simulink model "nucleo_g431re_ihm07m1"  (R2024a)
settings: Solver=FixedStepDiscrete  StartTime=0.0  StopTime=10  FixedStep=Ts  RelTol=1e-3  EnableMultiTasking=on
model workspace (MAT data in the model file):
  encoderResolution = 2000
  hallOffset = '0.5'
  indexOffset = 850
  polePairs = '4'
values from neighbouring files (symbols this model uses):
  motorParam =     [matlab.mat]
  PWM_Counter_Period = round(CPU_frequency/PWM_frequency/2)    [mcb_stm32_param_est_InitFunc.m]
  Ts = 1/PWM_frequency    (= 5e-05)    [mcb_stm32_param_est_InitFunc.m]    (also in stm32_pmsm_foc_data.m)
undefined symbols (not defined in the file or in its folder): DiscIntNeverNeededParam, inverter, NumBits1, NumBits2, Slope1, Slope2
libraries: mcbcontrolslib x24, simulink x15, stm32f4xxblockslib x4, stm32g4xxblockslib x3, slpidlib x2, stm32blockslib x2, svdutilitieslib x1
(part 1 of 3)
settings Model: Creator=The MathWorks, Inc.  LastModifiedBy=wsl
settings SolverCC: AlgebraicLoopSolver=TrustRegion  AutoInsertRateTranBlk=on  MaxZcPerStep=1
settings DataIOCC: LimitDataPoints=on  SaveFormat=Array  SaveOutput=off  SaveTime=off  ReturnWorkspaceOutputs=off
settings OptimizationCC: DefaultParameterBehavior=Inlined  DefaultUnderspecifiedDataType=single  InlineInvariantSignals=on  OptimizeBlockIOStorage=off  BufferReuse=off  ReuseModelBlockBuffer=off  GlobalBufferReuse=off  ExpressionFolding=off  ExpressionDepthLimit=2147483647  LocalBlockOutputs=off  ZeroExternalMemoryAtStartup=off  InitFltsAndDblsToZero=on  NoFixptDivByZeroProtection=on  EfficientFloat2IntCast=on  EfficientMapNaN2IntZero=off  LifeSpan=Inf  MaxStackSize=1024  OptimizeDataStoreBuffers=off  BusAssignmentInplaceUpdate=off  EfficientTunableParamExpr=on
settings DebuggingCC: ReadBeforeWriteMsg=DisableAll  WriteAfterWriteMsg=DisableAll  WriteAfterReadMsg=DisableAll  CheckSSInitialOutputMsg=off  SignalResolutionControl=TryResolveAllWithWarning  SolverPrmCheckMsg=warning  InheritedTsInSrcMsg=none  MultiTaskDSMMsg=none  MultiTaskCondExecSysMsg=none  TasksWithSamePriorityMsg=none  SigSpecEnsureSampleTimeMsg=none  IntegerOverflowMsg=none  ParameterPrecisionLossMsg=none  FcnCallInpInsideContextMsg=warning  UnconnectedInputMsg=warning  UnconnectedOutputMsg=warning  UnconnectedLineMsg=warning  AllowSymbolicDim=off  StateNameClashWarn=warning  SubsystemReferenceDiagnosticForUnitTest=warning  SFUnexpectedBacktrackingDiag=warning  SFNoUnconditionalDefaultTransitionDiag=warning  SFExecutionAtInitializationDiag=none  IntegerSaturationMsg=none  ArithmeticOperatorsInVariantConditions=warning
settings HardwareCC: ProdBitPerPointer=32  ProdBitPerSizeT=32  ProdBitPerPtrDiffT=32  ProdLargestAtomicInteger=Long  ProdLargestAtomicFloat=Double  ProdWordSize=32  ProdLongLongMode=on  ProdHWDeviceType=ARM Compatible->ARM Cortex  TargetBitPerChar=16  TargetBitPerInt=16  TargetBitPerPointer=16  TargetLargestAtomicInteger=Integer  TargetIntDivRoundTo=Zero  TargetEndianess=LittleEndian  TargetWordSize=16  TargetHWDeviceType=TI C2000
settings ModelReferenceCC: EnableRefExpFcnMdlSchedulingChecks=on  PropagateSignalLabelsOutOfModel=off
settings SFSimCC: SimUseLocalCustomCode=off  MATLABDynamicMemAlloc=off  CustomCodeUndefinedFunction=UseInterfaceOnly
settings RTWCC: Description=Embedded Coder  SystemTargetFile=ert.tlc  HardwareBoard=STM32G4xx Based  TemplateMakefile=ert_default_tmf  GenerateReport=on  RTWUseLocalCustomCode=off  Toolchain=GNU Tools for ARM Embedded Processors  BuildConfiguration=Faster Runs  IncludeHyperlinkInReport=on  LaunchReport=on  GenerateTraceInfo=on  GenerateTraceReport=on  GenerateTraceReportSl=on  GenerateTraceReportSf=on  GPUComputeCapability=3.5  DLArmComputeVersion=19.05
settings CodeAppCC: IgnoreCustomStorageClasses=off  CustomSymbolStrType=$N$R$M  StateflowObjectComments=on  InternalIdentifier=Classic
settings ERTTargetCC: TargetLangStandard=C99 (ISO)  CodeReplacementLibrary=ARM Cortex-M  MultiwordLength=2048  ExtModeTransport=3  ExtModeStaticAlloc=on  ExtModeStaticAllocSize=2048  ExtModeMexFile=ext_xcp  ExtModeIntrfLevel=Level2 - Open  ConvertIfToSwitch=off  SuppressUnreachableDefaultCases=off  MemSecPackage=tic2000demospkg
settings ConfigComp: CovMetricSettings=dw  CovSaveCumulativeToWorkspaceVar=on  CovSaveSingleToWorkspaceVar=on  CovExternalEMLEnable=off  CovSFcnEnable=off

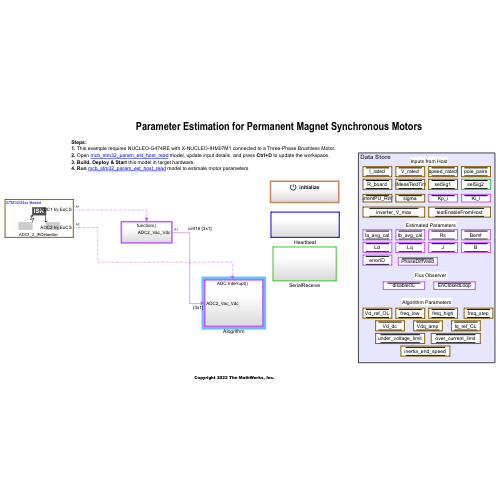
[thumbnail: Simulink's stored preview of the top-level diagram]
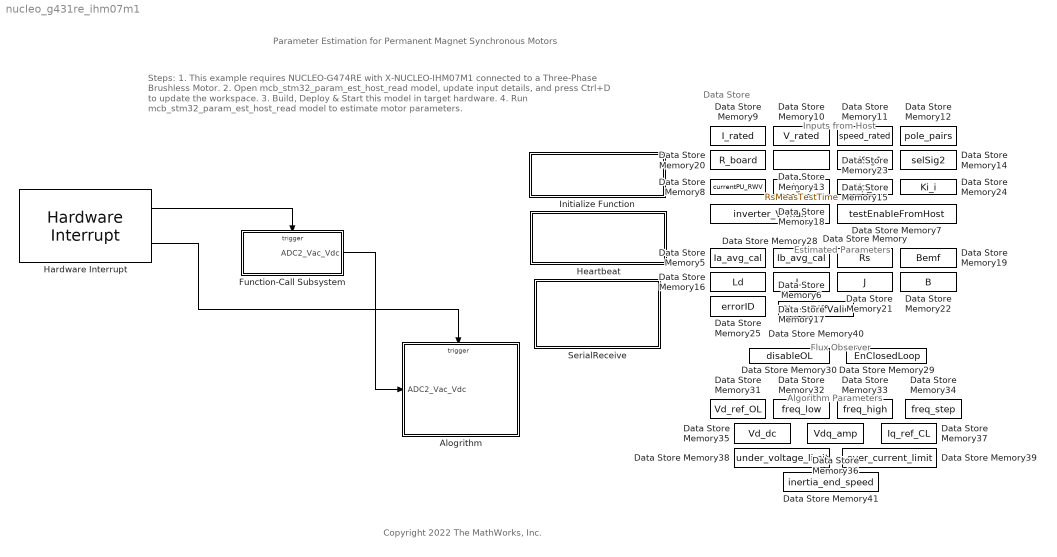
== system nucleo_g431re_ihm07m1 ==
  note: Flux Observer
  note: Estimated Parameters
  note: Data Store
  note: Inputs from Host
  note: Parameter Estimation for Permanent Magnet Synchronous Motors
  note: Steps:
      | 1. This example requires NUCLEO-G474RE with X-NUCLEO-IHM07M1 connected to a Three-Phase Brushless Motor.
      | 2. Open mcb_stm32_param_est_host_read model, update input details, and press Ctrl+D to update the workspace.
      | 3. Build, Deploy & Start this model in target hardware.
      | 4. Run mcb_stm32_param_est_host_read model to estimate motor parameters.
  note: Algorithm Parameters
  note: Copyright 2022 The MathWorks, Inc.
  Alogrithm : Subsystem
  Data Store Memory : DataStoreMemory  DataStoreName=Rs  ReadBeforeWriteMsg=warning  WriteAfterWriteMsg=warning  WriteAfterReadMsg=warning  InitialValue=1  ShowAdditionalParam=off  OutDataTypeStr=single
  Data Store Memory10 : DataStoreMemory  DataStoreName=V_rated  ReadBeforeWriteMsg=warning  WriteAfterWriteMsg=warning  WriteAfterReadMsg=warning  InitialValue=1  ShowAdditionalParam=off  OutDataTypeStr=single
  Data Store Memory11 : DataStoreMemory  DataStoreName=speed_rated  ReadBeforeWriteMsg=warning  WriteAfterWriteMsg=warning  WriteAfterReadMsg=warning  InitialValue=1  ShowAdditionalParam=off  OutDataTypeStr=single
  Data Store Memory12 : DataStoreMemory  DataStoreName=pole_pairs  ReadBeforeWriteMsg=warning  WriteAfterWriteMsg=warning  WriteAfterReadMsg=warning  InitialValue=1  ShowAdditionalParam=off  OutDataTypeStr=single
  Data Store Memory13 : DataStoreMemory  DataStoreName=RsMeasTestTime  ReadBeforeWriteMsg=warning  WriteAfterWriteMsg=warning  WriteAfterReadMsg=warning  InitialValue=1  ShowAdditionalParam=off  OutDataTypeStr=single
  Data Store Memory14 : DataStoreMemory  DataStoreName=selSig2  ReadBeforeWriteMsg=warning  WriteAfterWriteMsg=warning  WriteAfterReadMsg=warning  InitialValue=1  ShowAdditionalParam=off  OutDataTypeStr=single
  Data Store Memory15 : DataStoreMemory  DataStoreName=selSig1  ReadBeforeWriteMsg=warning  WriteAfterWriteMsg=warning  WriteAfterReadMsg=warning  InitialValue=1  ShowAdditionalParam=off  OutDataTypeStr=single
  Data Store Memory16 : DataStoreMemory  DataStoreName=Ld  ReadBeforeWriteMsg=warning  WriteAfterWriteMsg=warning  WriteAfterReadMsg=warning  InitialValue=1  ShowAdditionalParam=off
  Data Store Memory17 : DataStoreMemory  DataStoreName=Lq  ReadBeforeWriteMsg=warning  WriteAfterWriteMsg=warning  WriteAfterReadMsg=warning  InitialValue=1  ShowAdditionalParam=off
  Data Store Memory18 : DataStoreMemory  DataStoreName=sigma  ReadBeforeWriteMsg=warning  WriteAfterWriteMsg=warning  WriteAfterReadMsg=warning  InitialValue=1  ShowAdditionalParam=off  OutDataTypeStr=single
  Data Store Memory19 : DataStoreMemory  DataStoreName=Bemf  ReadBeforeWriteMsg=warning  WriteAfterWriteMsg=warning  WriteAfterReadMsg=warning  InitialValue=1  ShowAdditionalParam=off
  Data Store Memory20 : DataStoreMemory  DataStoreName=R_board  ReadBeforeWriteMsg=warning  WriteAfterWriteMsg=warning  WriteAfterReadMsg=warning  InitialValue=1  ShowAdditionalParam=off
  Data Store Memory21 : DataStoreMemory  DataStoreName=J  ReadBeforeWriteMsg=warning  WriteAfterWriteMsg=warning  WriteAfterReadMsg=warning  InitialValue=1  ShowAdditionalParam=off
  Data Store Memory22 : DataStoreMemory  DataStoreName=B  ReadBeforeWriteMsg=warning  WriteAfterWriteMsg=warning  WriteAfterReadMsg=warning  InitialValue=1  ShowAdditionalParam=off
  Data Store Memory23 : DataStoreMemory  DataStoreName=Kp_i  ReadBeforeWriteMsg=warning  WriteAfterWriteMsg=warning  WriteAfterReadMsg=warning  ShowAdditionalParam=off  OutDataTypeStr=single
  Data Store Memory24 : DataStoreMemory  DataStoreName=Ki_i  ReadBeforeWriteMsg=warning  WriteAfterWriteMsg=warning  WriteAfterReadMsg=warning  ShowAdditionalParam=off  OutDataTypeStr=single
  Data Store Memory25 : DataStoreMemory  DataStoreName=errorID  ReadBeforeWriteMsg=warning  WriteAfterWriteMsg=warning  WriteAfterReadMsg=warning  ShowAdditionalParam=off
  Data Store Memory28 : DataStoreMemory  DataStoreName=inverter_V_max  ReadBeforeWriteMsg=warning  WriteAfterWriteMsg=warning  WriteAfterReadMsg=warning  InitialValue=1  ShowAdditionalParam=off  OutDataTypeStr=single
  Data Store Memory29 : DataStoreMemory  DataStoreName=EnClosedLoop  ReadBeforeWriteMsg=warning  WriteAfterWriteMsg=warning  WriteAfterReadMsg=warning  ShowAdditionalParam=off
  Data Store Memory30 : DataStoreMemory  DataStoreName=disableOL  ReadBeforeWriteMsg=warning  WriteAfterWriteMsg=warning  WriteAfterReadMsg=warning  InitialValue=1  ShowAdditionalParam=off
  Data Store Memory31 : DataStoreMemory  DataStoreName=Vd_ref_OL  ReadBeforeWriteMsg=warning  WriteAfterWriteMsg=warning  WriteAfterReadMsg=warning  InitialValue=0.1  ShowAdditionalParam=off  OutDataTypeStr=single
  Data Store Memory32 : DataStoreMemory  DataStoreName=freq_low  ReadBeforeWriteMsg=warning  WriteAfterWriteMsg=warning  WriteAfterReadMsg=warning  InitialValue=400  ShowAdditionalParam=off  OutDataTypeStr=single
  Data Store Memory33 : DataStoreMemory  DataStoreName=freq_high  ReadBeforeWriteMsg=warning  WriteAfterWriteMsg=warning  WriteAfterReadMsg=warning  InitialValue=1000  ShowAdditionalParam=off  OutDataTypeStr=single
  Data Store Memory34 : DataStoreMemory  DataStoreName=freq_step  ReadBeforeWriteMsg=warning  WriteAfterWriteMsg=warning  WriteAfterReadMsg=warning  InitialValue=10  ShowAdditionalParam=off  OutDataTypeStr=single
  Data Store Memory35 : DataStoreMemory  DataStoreName=Vd_dc  ReadBeforeWriteMsg=warning  WriteAfterWriteMsg=warning  WriteAfterReadMsg=warning  InitialValue=0.1  ShowAdditionalParam=off  OutDataTypeStr=single
  Data Store Memory36 : DataStoreMemory  DataStoreName=Vdq_amp  ReadBeforeWriteMsg=warning  WriteAfterWriteMsg=warning  WriteAfterReadMsg=warning  InitialValue=0.05  ShowAdditionalParam=off  OutDataTypeStr=single
  Data Store Memory37 : DataStoreMemory  DataStoreName=Iq_ref_CL  ReadBeforeWriteMsg=warning  WriteAfterWriteMsg=warning  WriteAfterReadMsg=warning  InitialValue=0.2  ShowAdditionalParam=off  OutDataTypeStr=single
  Data Store Memory38 : DataStoreMemory  DataStoreName=under_voltage_limit  ReadBeforeWriteMsg=warning  WriteAfterWriteMsg=warning  WriteAfterReadMsg=warning  InitialValue=0.8  ShowAdditionalParam=off  OutDataTypeStr=single
  Data Store Memory39 : DataStoreMemory  DataStoreName=over_current_limit  ReadBeforeWriteMsg=warning  WriteAfterWriteMsg=warning  WriteAfterReadMsg=warning  InitialValue=1  ShowAdditionalParam=off  OutDataTypeStr=single
  Data Store Memory40 : DataStoreMemory  DataStoreName=PhaseDiffValid  ReadBeforeWriteMsg=warning  WriteAfterWriteMsg=warning  WriteAfterReadMsg=warning  ShowAdditionalParam=off
  Data Store Memory41 : DataStoreMemory  DataStoreName=inertia_end_speed  ReadBeforeWriteMsg=warning  WriteAfterWriteMsg=warning  WriteAfterReadMsg=warning  InitialValue=0.25  ShowAdditionalParam=off  OutDataTypeStr=single
  Data Store Memory5 : DataStoreMemory  DataStoreName=Ia_avg_cal  ReadBeforeWriteMsg=warning  WriteAfterWriteMsg=warning  WriteAfterReadMsg=warning  InitialValue=1  ShowAdditionalParam=off  OutDataTypeStr=single
  Data Store Memory6 : DataStoreMemory  DataStoreName=Ib_avg_cal  ReadBeforeWriteMsg=warning  WriteAfterWriteMsg=warning  WriteAfterReadMsg=warning  InitialValue=1  ShowAdditionalParam=off  OutDataTypeStr=single
  Data Store Memory7 : DataStoreMemory  DataStoreName=testEnableFromHost  ReadBeforeWriteMsg=warning  WriteAfterWriteMsg=warning  WriteAfterReadMsg=warning  InitialValue=1  ShowAdditionalParam=off  OutDataTypeStr=single
  Data Store Memory8 : DataStoreMemory  DataStoreName=currentPU_RWV  ReadBeforeWriteMsg=warning  WriteAfterWriteMsg=warning  WriteAfterReadMsg=warning  InitialValue=0.1  ShowAdditionalParam=off  OutDataTypeStr=single
  Data Store Memory9 : DataStoreMemory  DataStoreName=I_rated  ReadBeforeWriteMsg=warning  WriteAfterWriteMsg=warning  WriteAfterReadMsg=warning  InitialValue=1  ShowAdditionalParam=off  OutDataTypeStr=single
  Function-Call Subsystem : Subsystem  TreatAsAtomicUnit=on
  Hardware Interrupt : stm32g4xxblockslib/Hardware Interrupt  ISRGroup=Analog to digital converter (ADC)  ISRName=ADC1_2_IRQHandler  ISRNumber=33  EventsList={ 'off', 'ADC1 OVR', '1'; 'off', 'ADC1 Reg EoCS', '2'; 'on', 'ADC1 Inj EoCS', '2'; 'off', 'ADC1 Inj JQOVF', '4'; 'off', 'ADC1 Watchdog1', '5'; 'off', 'ADC1 Watchdog2', '6'; 'off', 'ADC1 Watchdog3', '7'; 'off', 'ADC2 OVR', '8'; 'off', 'ADC2 Reg EoCS', '9'; 'on', 'ADC2 Inj EoCS', '10'; 'off', 'ADC2 Inj JQOVF', '11'; 'off', 'ADC2 Watchdog', '12'; 'off', 'ADC2 Watchdog2', '13'; 'off', 'ADC2 Watchdog3', '14'; 'off', 'Custom event', '15' }  SelectedEvents={'ADC1 Inj EoCS','ADC2 Inj EoCS'}  TaskPriority=30  DisablePreemption=off  ClearInterruptFlagsAtEndOfEvent=off  InterruptDefinitionFile=$(TARGET_ROOT)/registry/interrupts/STM32F4xxBased_interrupts.xml  HardwareBoard=STM32G4xx Based  EnableSimPort=off
  Heartbeat : Subsystem
  Initialize Function : Subsystem  TreatAsAtomicUnit=on
  SerialReceive : Subsystem  SystemSampleTime=1e-3
  wires:
  Hardware Interrupt/2 -> Alogrithm/Trigger
  Hardware Interrupt/1 -> Function-Call Subsystem/Trigger
  Function-Call Subsystem/1(ADC2_Vac_Vdc) -> Alogrithm/1(ADC2_Vac_Vdc)

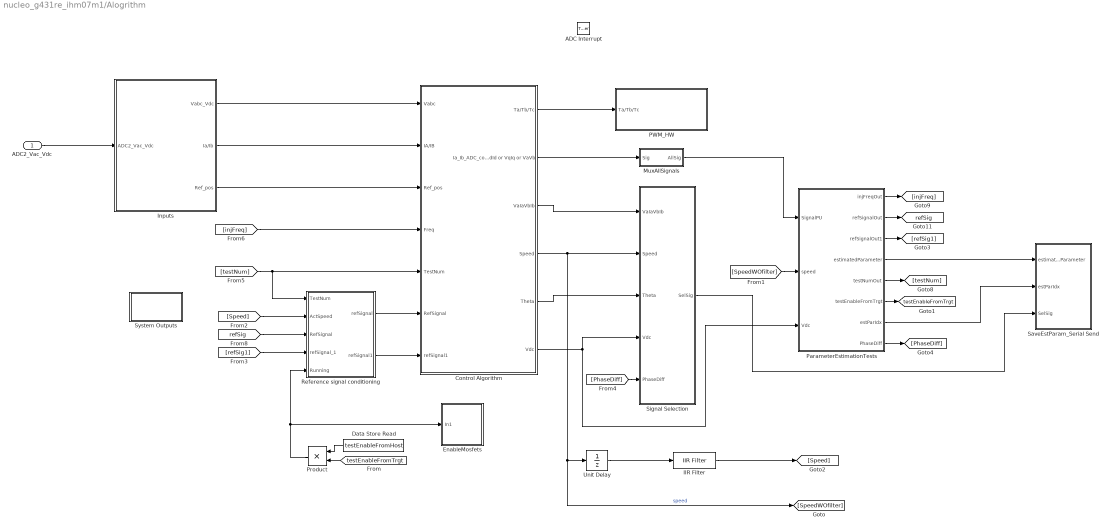
== system nucleo_g431re_ihm07m1/Alogrithm ==
  ADC2_Vac_Vdc : Inport
  ADC Interrupt : TriggerPort  TriggerType=function-call  VariantControl=Variant
  Control Algorithm : Subsystem
  Data Store Read : DataStoreRead  DataStoreName=testEnableFromHost  IndexOptions=Index vector (dialog)  Indices=1  OutputSizes=1
  EnableMosfets : Subsystem
  IIR Filter : mcbcontrolslib/IIR Filter  VariantControl=Low Pass Filter  VariantSelect=Low-pass  FilterConstantInputType=Specify via dialog  Filter_constant=0.01*(Ts/(50e-6))  advancedSettings=off  Ts=50e-6  cutOff_freq=64.9612
  Inputs : Subsystem
  MuxAllSignals : Subsystem
  PWM_HW : Subsystem
  ParameterEstimationTests : Subsystem
  Product : Product  OutDataTypeStr=single
  Reference signal conditioning : Subsystem
  SaveEstParam_Serial Send : Subsystem
  Signal Selection : Subsystem
  System Outputs : Subsystem  mask(System Outputs){ShowInLibBrowser=0}
      mask prompts: ShowInLibBrowser "Simulink:masks:CustCodeMaskParam1_MP"
      settings: CopyFcn=cccopyfcn(gcb)  OpenFcn=ccopenfcn('System Outputs Function')
      mask Help: eval('feval(''rtwprivate'',''rtwhelpview'',''rtw_sys_outputs_block'')');
      mask Display: disp('System\nOutputs');
  Unit Delay : UnitDelay  SampleTime=-1  HasFrameUpgradeWarning=on
  tag scope: refSig=global, testEnableFromTrgt=global
  wires:
  Inputs/2(Ia/Ib) -> Control Algorithm/2(IA/IB)
  [testNum] -> Reference signal conditioning/1(TestNum), Control Algorithm/5(TestNum)
  Inputs/3("Ref_pos ") -> Control Algorithm/3(Ref_pos)
  [injFreq] -> Control Algorithm/4(Freq)
  Control Algorithm/2(Ia_Ib_ADC_count or VdId or VqIq or VaVb) -> MuxAllSignals/1(Sig)
  Control Algorithm/5(Theta) -> Signal Selection/3(Theta)
  Control Algorithm/3(VaIaVbIb) -> Signal Selection/1(VaIaVbIb)
  Inputs/1(Vabc_Vdc) -> Control Algorithm/1(Vabc)
  [Speed] -> Reference signal conditioning/2(ActSpeed)
  Control Algorithm/4(Speed) -> [SpeedWOfilter], Unit Delay/1, Signal Selection/2(Speed)  "speed"
  Control Algorithm/6(Vdc) -> ParameterEstimationTests/3(Vdc), Signal Selection/4(Vdc)
  ParameterEstimationTests/2(refSignalOut) -> [refSig]
  ParameterEstimationTests/1(injFreqOut) -> [injFreq]
  [refSig] -> Reference signal conditioning/3("RefSignal ")
  Product/1 -> Reference signal conditioning/5(Running), EnableMosfets/1(In1)
  ParameterEstimationTests/5(testNumOut) -> [testNum]
  Data Store Read/1 -> Product/1
  ParameterEstimationTests/6(testEnableFromTrgt) -> [testEnableFromTrgt]
  [testEnableFromTrgt] -> Product/2
  Unit Delay/1 -> IIR Filter/1
  IIR Filter/1 -> [Speed]
  [SpeedWOfilter] -> ParameterEstimationTests/2(speed)
  Signal Selection/1(SelSig) -> SaveEstParam_Serial Send/3(SelSig)
  MuxAllSignals/1(AllSig) -> ParameterEstimationTests/1(SignalPU)
  ParameterEstimationTests/4(estimatedParameter) -> SaveEstParam_Serial Send/1(estimatedParameter)
  ParameterEstimationTests/7(estParIdx) -> SaveEstParam_Serial Send/2(estParIdx)
  ParameterEstimationTests/3(refSignalOut1) -> [refSig1]
  [refSig1] -> Reference signal conditioning/4(refSignal_1)
  Reference signal conditioning/1(refSignal) -> Control Algorithm/6(RefSignal)
  Reference signal conditioning/2(refSignal1) -> Control Algorithm/7(refSignal1)
  ParameterEstimationTests/8(PhaseDiff) -> [PhaseDiff]
  [PhaseDiff] -> Signal Selection/5(PhaseDiff)
  ADC2_Vac_Vdc/1 -> Inputs/1(ADC2_Vac_Vdc)
  Control Algorithm/1(Ta/Tb/Tc) -> PWM_HW/1(Ta/Tb/Tc)

== system nucleo_g431re_ihm07m1/Function-Call Subsystem ==
  function : TriggerPort  TriggerType=function-call  VariantControl=(inherit)
  Analog to Digital Converter1 : stm32f4xxblockslib/Analog to Digital Converter  ADCModule=ADC2  ConversionGroup=Injected  TriggerMode=Read results only  NumberOfConversions=3  EnableBufferConv=off  BufferLength=1  OutputStatus=off  SampleTime=-1  EnableSimPort=off
  ADC2_Vac_Vdc : Outport
  wires:
  Analog to Digital Converter1/1 -> ADC2_Vac_Vdc/1

== system nucleo_g431re_ihm07m1/Heartbeat ==
  Digital Port Write : stm32f4xxblockslib/Digital Port Write  PortName=GPIOA  PinNumber=[5]  ReadOperation=off  IOAsArray=on  EnableSimPort=off
  NOT : Logic  Operator=NOT  IconShape=distinctive  AllPortsSameDT=off  OutDataTypeStr=boolean
  Unit Delay : UnitDelay  InitialCondition=false  SampleTime=0.5  HasFrameUpgradeWarning=on
  wires:
  Unit Delay/1 -> NOT/1, Digital Port Write/1
  NOT/1 -> Unit Delay/1

== system nucleo_g431re_ihm07m1/Initialize Function ==
  Constant : Constant  Value=PWM_Counter_Period  OutDataTypeStr=uint16  SampleTime=-1
  Event Listener : EventListener  DisableCoverage=on  EventName=reset
  PWM Output : stm32g4xxblockslib/PWM Output  TimerModule=TIM1  DutycycleUnits=Counts  EnableChannel1=off  EnableChannel2=off  EnableChannel3=off  EnableChannel4=off  EnableChannel5=off  EnableChannel6=off  EnableCounterInput=off  EnableMainOutputInput=off  EnableFrequencyInput=on  SetRCAfterCE=on  OutputDirection=off  OutputMainOutputEnableStatus=off  SampleTime=-1  EnableSimPort=off  EnableUpdateEvent=off  EnableCaptureCompare1Event=off  EnableCaptureCompare2Event=off  EnableCaptureCompare3Event=off  EnableCaptureCompare4Event=off  EnableTriggerEvent=off  EnableBreakEvent=off  EnableBreakEvent2=off  ProcessorFamily=STM32G4  hoistedMaskSrc=ECSoC/ECSimCodegen/PWM Output
  wires:
  Constant/1 -> PWM Output/1

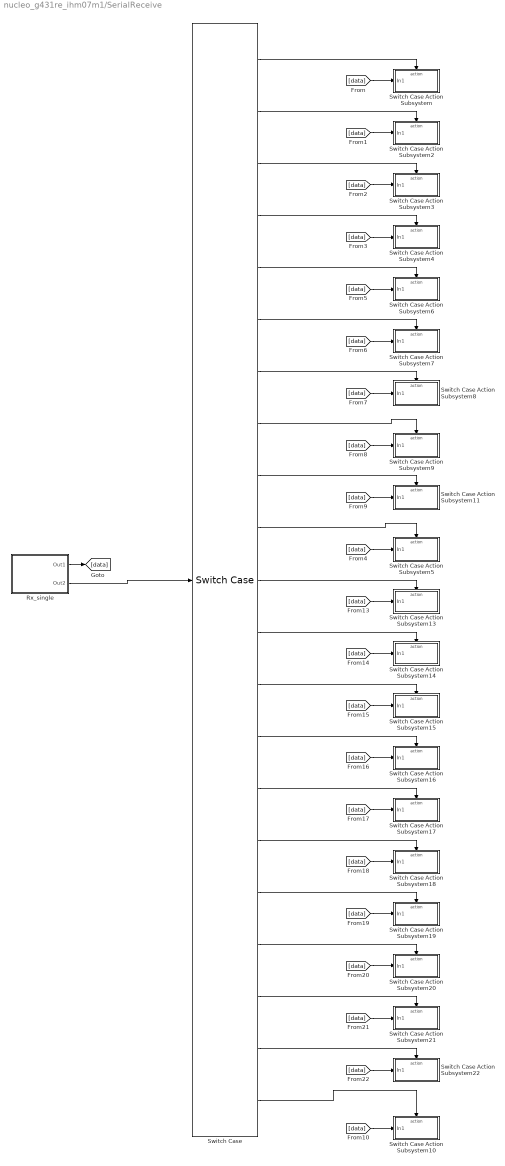
== system nucleo_g431re_ihm07m1/SerialReceive ==
  Rx_single : Subsystem
  Switch Case : SwitchCase  CaseConditions={1 2 3 4 5 6 7 8 9 10 13 14 15 16 17 18 19 20 21 22 23}  ShowDefaultCase=off
  Switch Case Action Subsystem : Subsystem  TreatAsAtomicUnit=on
  Switch Case Action Subsystem10 : Subsystem  TreatAsAtomicUnit=on
  Switch Case Action Subsystem11 : Subsystem  TreatAsAtomicUnit=on
  Switch Case Action Subsystem13 : Subsystem  TreatAsAtomicUnit=on
  Switch Case Action Subsystem14 : Subsystem  TreatAsAtomicUnit=on
  Switch Case Action Subsystem15 : Subsystem  TreatAsAtomicUnit=on
  Switch Case Action Subsystem16 : Subsystem  TreatAsAtomicUnit=on
  Switch Case Action Subsystem17 : Subsystem  TreatAsAtomicUnit=on
  Switch Case Action Subsystem18 : Subsystem  TreatAsAtomicUnit=on
  Switch Case Action Subsystem19 : Subsystem  TreatAsAtomicUnit=on
  Switch Case Action Subsystem2 : Subsystem  TreatAsAtomicUnit=on
  Switch Case Action Subsystem20 : Subsystem  TreatAsAtomicUnit=on
  Switch Case Action Subsystem21 : Subsystem  TreatAsAtomicUnit=on
  Switch Case Action Subsystem22 : Subsystem  TreatAsAtomicUnit=on
  Switch Case Action Subsystem3 : Subsystem  TreatAsAtomicUnit=on
  Switch Case Action Subsystem4 : Subsystem  TreatAsAtomicUnit=on
  Switch Case Action Subsystem5 : Subsystem  TreatAsAtomicUnit=on
  Switch Case Action Subsystem6 : Subsystem  TreatAsAtomicUnit=on
  Switch Case Action Subsystem7 : Subsystem  TreatAsAtomicUnit=on
  Switch Case Action Subsystem8 : Subsystem  TreatAsAtomicUnit=on
  Switch Case Action Subsystem9 : Subsystem  TreatAsAtomicUnit=on
  wires:
  Rx_single/1(Out1) -> [data]
  Switch Case/3 -> Switch Case Action Subsystem3/Action
  [data] -> Switch Case Action Subsystem22/1(In1)
  [data] -> Switch Case Action Subsystem4/1(In1)
  Switch Case/8 -> Switch Case Action Subsystem9/Action
  Switch Case/2 -> Switch Case Action Subsystem2/Action
  [data] -> Switch Case Action Subsystem15/1(In1)
  [data] -> Switch Case Action Subsystem2/1(In1)
  [data] -> Switch Case Action Subsystem20/1(In1)
  [data] -> Switch Case Action Subsystem14/1(In1)
  [data] -> Switch Case Action Subsystem21/1(In1)
  [data] -> Switch Case Action Subsystem16/1(In1)
  [data] -> Switch Case Action Subsystem6/1(In1)
  Switch Case/6 -> Switch Case Action Subsystem7/Action
  [data] -> Switch Case Action Subsystem18/1(In1)
  Switch Case/1 -> Switch Case Action Subsystem/Action
  Switch Case/4 -> Switch Case Action Subsystem4/Action
  [data] -> Switch Case Action Subsystem/1(In1)
  [data] -> Switch Case Action Subsystem10/1(In1)
  Switch Case/7 -> Switch Case Action Subsystem8/Action
  [data] -> Switch Case Action Subsystem5/1(In1)
  [data] -> Switch Case Action Subsystem11/1(In1)
  [data] -> Switch Case Action Subsystem8/1(In1)
  [data] -> Switch Case Action Subsystem9/1(In1)
  [data] -> Switch Case Action Subsystem7/1(In1)
  [data] -> Switch Case Action Subsystem3/1(In1)
  [data] -> Switch Case Action Subsystem17/1(In1)
  Switch Case/5 -> Switch Case Action Subsystem6/Action
  [data] -> Switch Case Action Subsystem13/1(In1)
  [data] -> Switch Case Action Subsystem19/1(In1)
  Switch Case/9 -> Switch Case Action Subsystem11/Action
  Switch Case/10 -> Switch Case Action Subsystem5/Action
  Switch Case/18 -> Switch Case Action Subsystem20/Action
  Switch Case/19 -> Switch Case Action Subsystem21/Action
  Switch Case/17 -> Switch Case Action Subsystem19/Action
  Switch Case/20 -> Switch Case Action Subsystem22/Action
  Switch Case/16 -> Switch Case Action Subsystem18/Action
  Switch Case/15 -> Switch Case Action Subsystem17/Action
  Switch Case/14 -> Switch Case Action Subsystem16/Action
  Switch Case/11 -> Switch Case Action Subsystem13/Action
  Switch Case/12 -> Switch Case Action Subsystem14/Action
  Switch Case/13 -> Switch Case Action Subsystem15/Action
  Switch Case/21 -> Switch Case Action Subsystem10/Action
  Rx_single/2(Out2) -> Switch Case/1

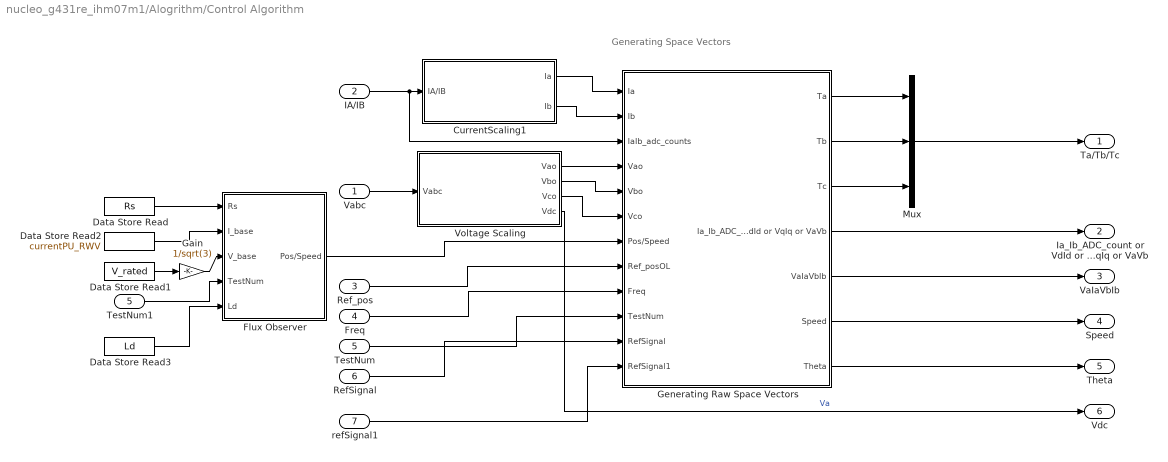
== system nucleo_g431re_ihm07m1/Alogrithm/Control Algorithm ==
  note: Generating Space Vectors
  Vabc : Inport
  IA/IB : Inport  Port=2
  Ref_pos : Inport  Port=3
  Freq : Inport  Port=4
  TestNum : Inport  Port=5
  RefSignal : Inport  Port=6
  refSignal1 : Inport  Port=7
  CurrentScaling1 : Subsystem
  Data Store Read : DataStoreRead  DataStoreName=Rs  IndexOptions=Index vector (dialog)  Indices=1  OutputSizes=1
  Data Store Read1 : DataStoreRead  DataStoreName=V_rated  IndexOptions=Index vector (dialog)  Indices=1  OutputSizes=1
  Data Store Read2 : DataStoreRead  DataStoreName=currentPU_RWV  IndexOptions=Index vector (dialog)  Indices=1  OutputSizes=1
  Data Store Read3 : DataStoreRead  DataStoreName=Ld  IndexOptions=Index vector (dialog)  Indices=1  OutputSizes=1
  Flux Observer : Subsystem
  Gain : Gain  Gain=1/sqrt(3)
  Generating Raw Space Vectors : Subsystem
  Mux : Mux  Inputs=3
  TestNum1 : InportShadow  Port=5
  Voltage Scaling : Subsystem
  Ta/Tb/Tc : Outport
  Ia_Ib_ADC_count or VdId or VqIq or VaVb : Outport  Port=2  OutDataTypeStr=single  VectorParamsAs1DForOutWhenUnconnected=off
  VaIaVbIb : Outport  Port=3  OutDataTypeStr=single  VectorParamsAs1DForOutWhenUnconnected=off
  Speed : Outport  Port=4  OutDataTypeStr=single  VectorParamsAs1DForOutWhenUnconnected=off
  Theta : Outport  Port=5  OutDataTypeStr=single  VectorParamsAs1DForOutWhenUnconnected=off
  Vdc : Outport  Port=6  OutDataTypeStr=single  VectorParamsAs1DForOutWhenUnconnected=off
  wires:
  Vabc/1 -> Voltage Scaling/1(Vabc)
  IA/IB/1 -> Generating Raw Space Vectors/3(IaIb_adc_counts), CurrentScaling1/1(IA/IB)
  Generating Raw Space Vectors/2(Tb) -> Mux/2
  Voltage Scaling/1(Vao) -> Generating Raw Space Vectors/4(Vao)
  Mux/1 -> Ta/Tb/Tc/1
  CurrentScaling1/2(Ib) -> Generating Raw Space Vectors/2(Ib)
  CurrentScaling1/1(Ia) -> Generating Raw Space Vectors/1(Ia)
  Generating Raw Space Vectors/3(Tc) -> Mux/3
  Generating Raw Space Vectors/1(Ta) -> Mux/1
  Ref_pos/1 -> Generating Raw Space Vectors/8(Ref_posOL)
  Freq/1 -> Generating Raw Space Vectors/9(Freq)
  TestNum/1 -> Generating Raw Space Vectors/10(TestNum)
  RefSignal/1 -> Generating Raw Space Vectors/11(RefSignal)
  Generating Raw Space Vectors/4(Ia_Ib_ADC_count or VdId or VqIq or VaVb) -> Ia_Ib_ADC_count or VdId or VqIq or VaVb/1
  Generating Raw Space Vectors/5(VaIaVbIb) -> VaIaVbIb/1
  Generating Raw Space Vectors/6(Speed) -> Speed/1
  Generating Raw Space Vectors/7(Theta) -> Theta/1
  Voltage Scaling/2(Vbo) -> Generating Raw Space Vectors/5(Vbo)
  Voltage Scaling/3(Vco) -> Generating Raw Space Vectors/6(Vco)
  Flux Observer/1(Pos/Speed) -> Generating Raw Space Vectors/7(Pos/Speed)
  Voltage Scaling/4(Vdc) -> Vdc/1  "Va"
  Data Store Read/1 -> Flux Observer/1(Rs)
  Data Store Read2/1 -> Flux Observer/2(I_base)
  Gain/1 -> Flux Observer/3(V_base)
  Data Store Read1/1 -> Gain/1
  TestNum1/1 -> Flux Observer/4(TestNum)
  Data Store Read3/1 -> Flux Observer/5(Ld)
  refSignal1/1 -> Generating Raw Space Vectors/12(RefSignal1)

== system nucleo_g431re_ihm07m1/Alogrithm/EnableMosfets ==
  In1 : Inport
  DRV8305 Reset : Constant  Value=0  OutDataTypeStr=uint16  SampleTime=-1
  DRV8305 Set : Constant  OutDataTypeStr=uint16  SampleTime=-1
  Digital Port Write : stm32f4xxblockslib/Digital Port Write  PortName=GPIOC  PinNumber=[10 11 12]  ReadOperation=off  IOAsArray=off  EnableSimPort=off
  Switch : Switch  Criteria=u2 ~= 0  SaturateOnIntegerOverflow=off  InputSameDT=off
  wires:
  Switch/1 -> Digital Port Write/3, Digital Port Write/2, Digital Port Write/1
  In1/1 -> Switch/2
  DRV8305 Reset/1 -> Switch/3
  DRV8305 Set/1 -> Switch/1

== system nucleo_g431re_ihm07m1/Alogrithm/Inputs ==
  ADC2_Vac_Vdc : Inport
  Analog to Digital Converter : stm32f4xxblockslib/Analog to Digital Converter  ADCModule=ADC1  ConversionGroup=Injected  TriggerMode=Read results only  NumberOfConversions=3  EnableBufferConv=off  BufferLength=1  OutputStatus=off  SampleTime=-1  EnableSimPort=off
  Demux : Demux  Outputs=3
  Demux1 : Demux  Outputs=3
  Mux : Mux
  Mux1 : Mux  Inputs=2
  Ref_pos : Constant  Value=0  OutDataTypeStr=single  SampleTime=-1
  Vabc_Vdc : Outport  VectorParamsAs1DForOutWhenUnconnected=off
  Ia/Ib : Outport  Port=2  VectorParamsAs1DForOutWhenUnconnected=off
  "Ref_pos " : Outport  Port=3  VectorParamsAs1DForOutWhenUnconnected=off
  wires:
  Ref_pos/1 -> "Ref_pos "/1
  Demux1/3 -> Mux/2
  Mux/1 -> Vabc_Vdc/1
  Demux/2 -> Mux/3
  Demux/1 -> Mux/1
  ADC2_Vac_Vdc/1 -> Demux/1
  Demux/3 -> Mux/4
  Analog to Digital Converter/1 -> Demux1/1
  Demux1/1 -> Mux1/1
  Demux1/2 -> Mux1/2
  Mux1/1 -> Ia/Ib/1

== system nucleo_g431re_ihm07m1/Alogrithm/MuxAllSignals ==
  Sig : Inport
  Demux : Demux  Outputs=2
  Demux1 : Demux  Outputs=2
  Demux2 : Demux  Outputs=2
  Mux : Mux  Inputs=6
  AllSig : Outport
  wires:
  Mux/1 -> AllSig/1
  Sig/1 -> Demux/1
  Demux/1 -> Mux/1
  Demux/2 -> Mux/2
  Demux1/2 -> Mux/4
  Demux1/1 -> Mux/3
  Demux2/1 -> Mux/5
  Demux2/2 -> Mux/6
  [VdId_32_Q17] -> Demux1/1
  [VqIq_32_Q17] -> Demux2/1

== system nucleo_g431re_ihm07m1/Alogrithm/PWM_HW ==
  Ta/Tb/Tc : Inport
  Demux : Demux  Outputs=3
  PWM Output : stm32g4xxblockslib/PWM Output  TimerModule=TIM1  DutycycleUnits=Counts  EnableChannel1=on  EnableChannel2=on  EnableChannel3=on  EnableChannel4=off  EnableChannel5=off  EnableChannel6=off  EnableCounterInput=off  EnableMainOutputInput=off  EnableFrequencyInput=off  SetRCAfterCE=on  OutputDirection=off  OutputMainOutputEnableStatus=off  SampleTime=0.1  EnableSimPort=off  EnableUpdateEvent=off  EnableCaptureCompare1Event=off  EnableCaptureCompare2Event=off  EnableCaptureCompare3Event=off  EnableCaptureCompare4Event=off  EnableTriggerEvent=off  EnableBreakEvent=off  EnableBreakEvent2=off  ProcessorFamily=STM32G4  hoistedMaskSrc=ECSoC/ECSimCodegen/PWM Output
  PWM scaling : Subsystem
  wires:
  PWM scaling/1(PWM A/B/C) -> Demux/1
  Demux/2 -> PWM Output/2
  Demux/3 -> PWM Output/3
  Demux/1 -> PWM Output/1
  Ta/Tb/Tc/1 -> PWM scaling/1(Ta/Tb/Tc)

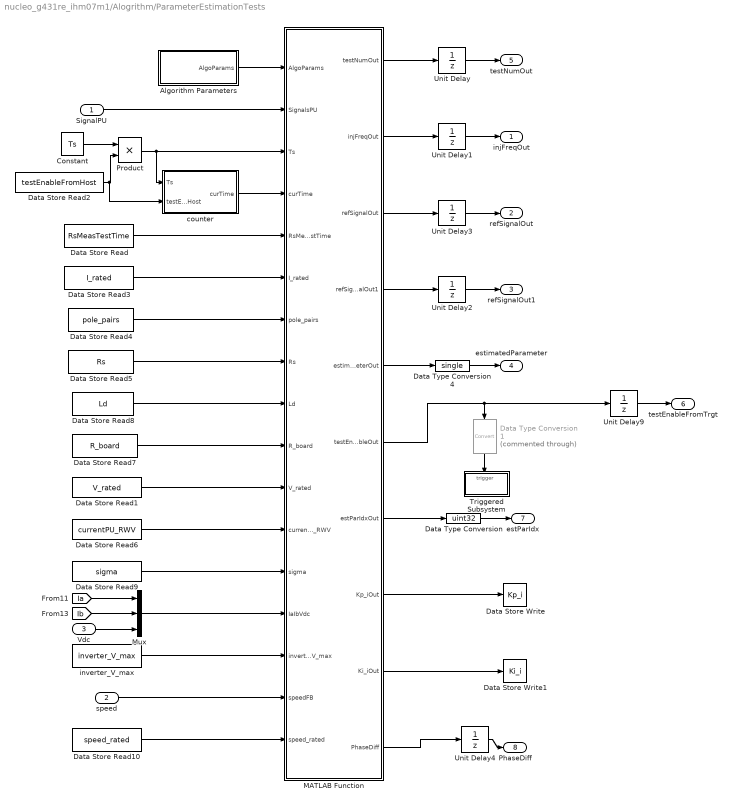
== system nucleo_g431re_ihm07m1/Alogrithm/ParameterEstimationTests ==
  SignalPU : Inport
  speed : Inport  Port=2
  Vdc : Inport  Port=3
  Algorithm Parameters : Subsystem
  Constant : Constant  Value=Ts  OutDataTypeStr=single  SampleTime=-1
  Data Store Read : DataStoreRead  DataStoreName=RsMeasTestTime  IndexOptions=Index vector (dialog)  Indices=1  OutputSizes=1
  Data Store Read1 : DataStoreRead  DataStoreName=V_rated  IndexOptions=Index vector (dialog)  Indices=1  OutputSizes=1
  Data Store Read10 : DataStoreRead  DataStoreName=speed_rated  IndexOptions=Index vector (dialog)  Indices=1  OutputSizes=1
  Data Store Read2 : DataStoreRead  DataStoreName=testEnableFromHost  IndexOptions=Index vector (dialog)  Indices=1  OutputSizes=1
  Data Store Read3 : DataStoreRead  DataStoreName=I_rated  IndexOptions=Index vector (dialog)  Indices=1  OutputSizes=1
  Data Store Read4 : DataStoreRead  DataStoreName=pole_pairs  IndexOptions=Index vector (dialog)  Indices=1  OutputSizes=1
  Data Store Read5 : DataStoreRead  DataStoreName=Rs  IndexOptions=Index vector (dialog)  Indices=1  OutputSizes=1
  Data Store Read6 : DataStoreRead  DataStoreName=currentPU_RWV  IndexOptions=Index vector (dialog)  Indices=1  OutputSizes=1
  Data Store Read7 : DataStoreRead  DataStoreName=R_board  IndexOptions=Index vector (dialog)  Indices=1  OutputSizes=1
  Data Store Read8 : DataStoreRead  DataStoreName=Ld  IndexOptions=Index vector (dialog)  Indices=1  OutputSizes=1
  Data Store Read9 : DataStoreRead  DataStoreName=sigma  IndexOptions=Index vector (dialog)  Indices=1  OutputSizes=1
  Data Store Write : DataStoreWrite  DataStoreName=Kp_i  IndexOptions=Index vector (dialog)  Indices=1  OutputSizes=1
  Data Store Write1 : DataStoreWrite  DataStoreName=Ki_i  IndexOptions=Index vector (dialog)  Indices=1  OutputSizes=1
  Data Type Conversion : DataTypeConversion  OutDataTypeStr=uint32  RndMeth=Simplest  SaturateOnIntegerOverflow=off
  Data Type Conversion1 : DataTypeConversion  Commented=through  SaturateOnIntegerOverflow=off  RndMeth=Floor
  Data Type Conversion4 : DataTypeConversion  OutDataTypeStr=single  RndMeth=Simplest  SaturateOnIntegerOverflow=off
  MATLAB Function : MATLAB Function  TreatAsAtomicUnit=on
  Mux : Mux  Inputs=3
  Product : Product  OutDataTypeStr=single
  Triggered Subsystem : Subsystem  TreatAsAtomicUnit=on
  Unit Delay{,1..4} (5 alike) : UnitDelay  SampleTime=-1  HasFrameUpgradeWarning=on
  Unit Delay9 : UnitDelay  InitialCondition=1  SampleTime=-1  HasFrameUpgradeWarning=on
  counter : Subsystem
  inverter_V_max : DataStoreRead  DataStoreName=inverter_V_max  IndexOptions=Index vector (dialog)  Indices=1  OutputSizes=1
  injFreqOut : Outport  InitialOutput=[0]
  refSignalOut : Outport  Port=2  InitialOutput=[0]
  refSignalOut1 : Outport  Port=3
  estimatedParameter : Outport  Port=4  InitialOutput=[0]
  testNumOut : Outport  Port=5  InitialOutput=[0]
  testEnableFromTrgt : Outport  Port=6  InitialOutput=[0]
  estParIdx : Outport  Port=7  InitialOutput=[0]
  PhaseDiff : Outport  Port=8
  wires:
  Data Store Read10/1 -> MATLAB Function/17(speed_rated)
  speed/1 -> MATLAB Function/16(speedFB)
  counter/1(curTime) -> MATLAB Function/4(curTime)
  Unit Delay2/1 -> refSignalOut1/1
  MATLAB Function/4(refSignalOut1) -> Unit Delay2/1
  MATLAB Function/10(PhaseDiff) -> Unit Delay4/1
  [Ib] -> Mux/2
  Algorithm Parameters/1(AlgoParams) -> MATLAB Function/1(AlgoParams)
  Data Type Conversion/1 -> estParIdx/1
  [Ia] -> Mux/1
  MATLAB Function/3(refSignalOut) -> Unit Delay3/1
  Data Type Conversion4/1 -> estimatedParameter/1
  Data Store Read9/1 -> MATLAB Function/13(sigma)
  Data Store Read4/1 -> MATLAB Function/7(pole_pairs)
  Unit Delay4/1 -> PhaseDiff/1
  MATLAB Function/2(injFreqOut) -> Unit Delay1/1
  Constant/1 -> Product/1
  MATLAB Function/7(estParIdxOut) -> Data Type Conversion/1
  MATLAB Function/1(testNumOut) -> Unit Delay/1
  Data Store Read2/1 -> counter/2(testEnableFromHost), Product/2
  Product/1 -> counter/1(Ts), MATLAB Function/3(Ts)
  MATLAB Function/5(estimatedParameterOut) -> Data Type Conversion4/1
  MATLAB Function/9(Ki_iOut) -> Data Store Write1/1
  Data Store Read/1 -> MATLAB Function/5(RsMeasTestTime)
  Unit Delay3/1 -> refSignalOut/1
  Data Store Read5/1 -> MATLAB Function/8(Rs)
  Data Store Read8/1 -> MATLAB Function/9(Ld)
  Mux/1 -> MATLAB Function/14(IaIbVdc)
  Data Store Read1/1 -> MATLAB Function/11(V_rated)
  MATLAB Function/6(testEnableOut) -> Unit Delay9/1, Data Type Conversion1/1
  Data Store Read7/1 -> MATLAB Function/10(R_board)
  Data Store Read3/1 -> MATLAB Function/6(I_rated)
  Data Store Read6/1 -> MATLAB Function/12(currentPU_RWV)
  Unit Delay9/1 -> testEnableFromTrgt/1
  Vdc/1 -> Mux/3
  MATLAB Function/8(Kp_iOut) -> Data Store Write/1
  inverter_V_max/1 -> MATLAB Function/15(inverter_V_max)
  Unit Delay/1 -> testNumOut/1
  SignalPU/1 -> MATLAB Function/2(SignalsPU)
  Unit Delay1/1 -> injFreqOut/1
  Data Type Conversion1/1 -> Triggered Subsystem/Trigger

== system nucleo_g431re_ihm07m1/Alogrithm/Reference signal conditioning ==
  TestNum : Inport
  ActSpeed : Inport  Port=2
  "RefSignal " : Inport  Port=3
  refSignal_1 : Inport  Port=4
  Running : Inport  Port=5
  Compare To Constant : simulink/Logic and Bit Operations/Compare To Constant  relop=>=  const=4  OutDataTypeStr=boolean
  Data Type Conversion3 : DataTypeConversion  OutDataTypeStr=single  SaturateOnIntegerOverflow=off  RndMeth=Floor
  Switch : Switch  Threshold=4  SaturateOnIntegerOverflow=off  InputSameDT=off
  TestNum1 : InportShadow
  Torque_control_with_speed_limit : Subsystem
  refSignal : Outport  VectorParamsAs1DForOutWhenUnconnected=off
  refSignal1 : Outport  Port=2
  wires:
  Switch/1 -> Data Type Conversion3/1
  TestNum/1 -> Switch/2
  Data Type Conversion3/1 -> refSignal/1
  "RefSignal "/1 -> Torque_control_with_speed_limit/1(MaxSpeed), Switch/3
  ActSpeed/1 -> Torque_control_with_speed_limit/3(ActSpeed)
  Running/1 -> Torque_control_with_speed_limit/4(En)
  Torque_control_with_speed_limit/1(Iq_ref) -> Switch/1
  Compare To Constant/1 -> Torque_control_with_speed_limit/Enable
  TestNum1/1 -> Compare To Constant/1
  refSignal_1/1 -> Torque_control_with_speed_limit/2(IqRef), refSignal1/1

== system nucleo_g431re_ihm07m1/Alogrithm/SaveEstParam_Serial Send ==
  estimatedParameter : Inport
  estParIdx : Inport  Port=2
  SelSig : Inport  Port=3
  ChangeDetect : Subsystem
  SaveToMemory : Subsystem
  Serial Send : Subsystem
  wires:
  estimatedParameter/1 -> ChangeDetect/1(Sig), SaveToMemory/1(estimatedParameter)
  SaveToMemory/1(Idx) -> Serial Send/1(Idx)
  SelSig/1 -> Serial Send/3(SelSig)
  SaveToMemory/2(EstPar) -> Serial Send/2(estimatedParameter)
  ChangeDetect/1(ChangeDet) -> SaveToMemory/Trigger
  estParIdx/1 -> SaveToMemory/2(estParIdx)

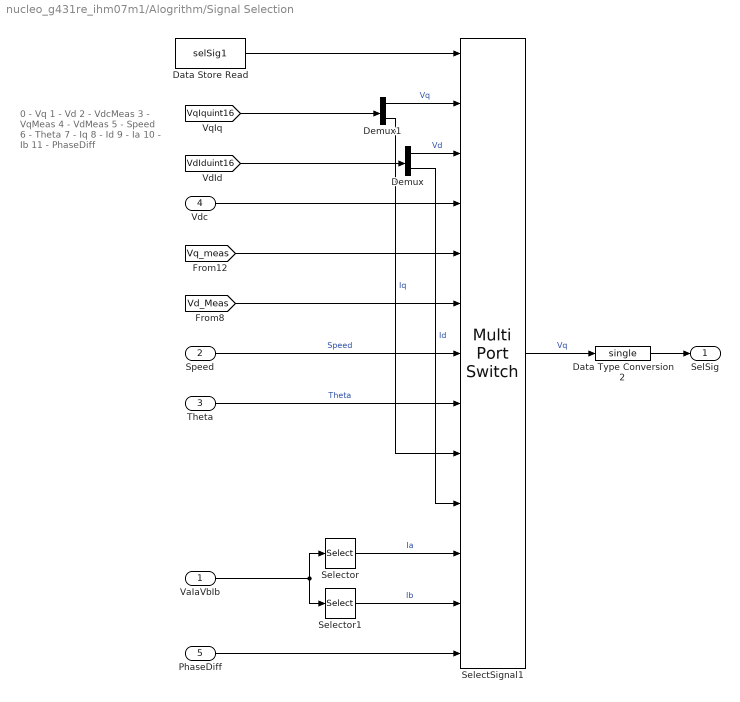
== system nucleo_g431re_ihm07m1/Alogrithm/Signal Selection ==
  note: 0 - Vq
      | 1 - Vd
      | 2 - VdcMeas
      | 3 - VqMeas
      | 4 - VdMeas
      | 5 - Speed
      | 6 - Theta
      | 7 - Iq
      | 8 - Id
      | 9 - Ia
      | 10 - Ib
      | 11 - PhaseDiff
  VaIaVbIb : Inport
  Speed : Inport  Port=2
  Theta : Inport  Port=3
  Vdc : Inport  Port=4
  PhaseDiff : Inport  Port=5
  Data Store Read : DataStoreRead  DataStoreName=selSig1  IndexOptions=Index vector (dialog)  Indices=1  OutputSizes=1
  Data Type Conversion2 : DataTypeConversion  OutDataTypeStr=single  RndMeth=Simplest  SaturateOnIntegerOverflow=off
  Demux : Demux  Outputs=2
  Demux1 : Demux  Outputs=2
  SelectSignal1 : MultiPortSwitch  DataPortOrder=Zero-based contiguous  Inputs=12  DiagnosticForDefault=None  zeroidx=on  SaturateOnIntegerOverflow=off  InputSameDT=off
  Selector : Selector  InputPortWidth=4  IndexOptions=Index vector (dialog)  Indices=[2]  OutputSizes=1
  Selector1 : Selector  InputPortWidth=4  IndexOptions=Index vector (dialog)  Indices=[4]  OutputSizes=1
  SelSig : Outport  VectorParamsAs1DForOutWhenUnconnected=off
  wires:
  Data Store Read/1 -> SelectSignal1/1
  VaIaVbIb/1 -> Selector/1, Selector1/1
  [VqIquint16] -> Demux1/1
  [VdIduint16] -> Demux/1
  Demux1/1 -> SelectSignal1/2  "Vq"
  Demux/1 -> SelectSignal1/3  "Vd"
  Speed/1 -> SelectSignal1/7  "Speed"
  Demux1/2 -> SelectSignal1/9  "Iq"
  Demux/2 -> SelectSignal1/10  "Id"
  Selector/1 -> SelectSignal1/11  "Ia"
  Selector1/1 -> SelectSignal1/12  "Ib"
  Theta/1 -> SelectSignal1/8  "Theta"
  [Vq_meas] -> SelectSignal1/5
  Data Type Conversion2/1 -> SelSig/1
  SelectSignal1/1 -> Data Type Conversion2/1  "Vq"
  Vdc/1 -> SelectSignal1/4
  [Vd_Meas] -> SelectSignal1/6
  PhaseDiff/1 -> SelectSignal1/13

== system nucleo_g431re_ihm07m1/Alogrithm/System Outputs ==

== system nucleo_g431re_ihm07m1/SerialReceive/Rx_single ==
  Compare To Zero : simulink/Logic and Bit Operations/Compare To Zero  relop===  OutDataTypeStr=boolean
  Data Type Conversion2 : DataTypeConversion  OutDataTypeStr=uint32  RndMeth=Simplest  SaturateOnIntegerOverflow=off
  Demux : Demux  Outputs=2
  Enabled Subsystem : Subsystem  TreatAsAtomicUnit=on
  UART/USART Read : stm32blockslib/UART//USART Read  Priority=2  UARTModule=LPUART1  DataType=single  DataLength=2  BlockingMode=off  BlockingTimeout=0.1  OutputLength=off  OutputStatus=on  SampleTime=1e-3/2
  Out1 : Outport
  Out2 : Outport  Port=2
  wires:
  Demux/2 -> Data Type Conversion2/1
  UART/USART Read/1 -> Enabled Subsystem/1(In1)
  UART/USART Read/2 -> Compare To Zero/1
  Compare To Zero/1 -> Enabled Subsystem/Enable
  Enabled Subsystem/1(Out1) -> Demux/1
  Demux/1 -> Out1/1
  Data Type Conversion2/1 -> Out2/1

== system nucleo_g431re_ihm07m1/SerialReceive/Switch Case Action Subsystem ==
  In1 : Inport
  Action Port : ActionPort  ActionPortLabel=case [ 1 ]:
  ADC_Gain_Setting : Constant  Priority=1000  Value=0x502A  OutDataTypeStr=uint16  SampleTime=-1
  ADC_Gain_Setting1 : Constant  Priority=1000  Value=0x5015  OutDataTypeStr=uint16  SampleTime=-1
  ADC_Gain_Setting2 : Constant  Priority=1000  Value=0x5000  OutDataTypeStr=uint16  SampleTime=-1
  Compare To Constant : simulink/Logic and Bit Operations/Compare To Constant  relop=>=  const=0  OutDataTypeStr=boolean
  Compare To Constant1 : simulink/Logic and Bit Operations/Compare To Constant  relop=>  const=5  OutDataTypeStr=boolean
  Compare To Constant2 : simulink/Logic and Bit Operations/Compare To Constant  relop=>  const=7  OutDataTypeStr=boolean
  Data Store Write1 : DataStoreWrite  DataStoreName=I_rated  IndexOptions=Index vector (dialog)  Indices=1  OutputSizes=1
  Display1 : Display
      settings: Format=hex (Stored Integer)
  Multiport Switch : MultiPortSwitch  SaturateOnIntegerOverflow=off  InputSameDT=off
  Sum : Sum  Inputs=+|+|+
  wires:
  ADC_Gain_Setting1/1 -> Multiport Switch/3
  Sum/1 -> Multiport Switch/1
  ADC_Gain_Setting2/1 -> Multiport Switch/4
  ADC_Gain_Setting/1 -> Multiport Switch/2
  Compare To Constant/1 -> Sum/1
  In1/1 -> Compare To Constant/1, Compare To Constant1/1, Compare To Constant2/1, Data Store Write1/1
  Multiport Switch/1 -> Display1/1
  Compare To Constant2/1 -> Sum/3
  Compare To Constant1/1 -> Sum/2

== system nucleo_g431re_ihm07m1/SerialReceive/Switch Case Action Subsystem10 ==
  In1 : Inport
  Action Port : ActionPort  ActionPortLabel=case [ 23 ]:
  Data Store Write1 : DataStoreWrite  DataStoreName=selSig1  IndexOptions=Index vector (dialog)  Indices=1  OutputSizes=1
  Data Store Write2 : DataStoreWrite  DataStoreName=selSig2  IndexOptions=Index vector (dialog)  Indices=1  OutputSizes=1
  Data Store Write3 : DataStoreWrite  DataStoreName=testEnableFromHost  IndexOptions=Index vector (dialog)  Indices=1  OutputSizes=1
  Data Type Conversion : DataTypeConversion  OutDataTypeStr=uint32  RndMeth=Simplest  SaturateOnIntegerOverflow=off
  bytepack : Subsystem
  wires:
  In1/1 -> Data Type Conversion/1
  Data Type Conversion/1 -> bytepack/1(testEnable_sigSel1_2)
  bytepack/1(testEnable) -> Data Store Write3/1
  bytepack/3(DetectParam2) -> Data Store Write2/1
  bytepack/2(DetectParam1) -> Data Store Write1/1

== system nucleo_g431re_ihm07m1/SerialReceive/Switch Case Action Subsystem11 ==
  In1 : Inport
  Action Port : ActionPort  ActionPortLabel=case [ 9 ]:
  Data Store Write3 : DataStoreWrite  Commented=on  DataStoreName=Position_offset  IndexOptions=Index vector (dialog)  Indices=1  OutputSizes=1
  wires:
  In1/1 -> Data Store Write3/1

== system nucleo_g431re_ihm07m1/SerialReceive/Switch Case Action Subsystem13 ==
  In1 : Inport
  Action Port : ActionPort  ActionPortLabel=case [ 13 ]:
  Data Store Write : DataStoreWrite  DataStoreName=Vd_ref_OL  IndexOptions=Index vector (dialog)  Indices=1  OutputSizes=1
  Saturation : Saturate  LowerLimit=0.01
  wires:
  In1/1 -> Saturation/1
  Saturation/1 -> Data Store Write/1

== system nucleo_g431re_ihm07m1/SerialReceive/Switch Case Action Subsystem14 ==
  In1 : Inport
  Action Port : ActionPort  ActionPortLabel=case [ 14 ]:
  Data Store Write : DataStoreWrite  DataStoreName=freq_low  IndexOptions=Index vector (dialog)  Indices=1  OutputSizes=1
  wires:
  In1/1 -> Data Store Write/1

== system nucleo_g431re_ihm07m1/SerialReceive/Switch Case Action Subsystem15 ==
  In1 : Inport
  Action Port : ActionPort  ActionPortLabel=case [ 15 ]:
  Data Store Write : DataStoreWrite  DataStoreName=freq_high  IndexOptions=Index vector (dialog)  Indices=1  OutputSizes=1
  wires:
  In1/1 -> Data Store Write/1

== system nucleo_g431re_ihm07m1/SerialReceive/Switch Case Action Subsystem16 ==
  In1 : Inport
  Action Port : ActionPort  ActionPortLabel=case [ 16 ]:
  Data Store Write : DataStoreWrite  DataStoreName=freq_step  IndexOptions=Index vector (dialog)  Indices=1  OutputSizes=1
  wires:
  In1/1 -> Data Store Write/1

== system nucleo_g431re_ihm07m1/SerialReceive/Switch Case Action Subsystem17 ==
  In1 : Inport
  Action Port : ActionPort  ActionPortLabel=case [ 17 ]:
  Data Store Write : DataStoreWrite  DataStoreName=Vd_dc  IndexOptions=Index vector (dialog)  Indices=1  OutputSizes=1
  Saturation : Saturate  LowerLimit=0.01
  wires:
  In1/1 -> Saturation/1
  Saturation/1 -> Data Store Write/1

== system nucleo_g431re_ihm07m1/SerialReceive/Switch Case Action Subsystem18 ==
  In1 : Inport
  Action Port : ActionPort  ActionPortLabel=case [ 18 ]:
  Data Store Write : DataStoreWrite  DataStoreName=Vdq_amp  IndexOptions=Index vector (dialog)  Indices=1  OutputSizes=1
  Saturation : Saturate  UpperLimit=0.9  LowerLimit=1e-3
  wires:
  In1/1 -> Saturation/1
  Saturation/1 -> Data Store Write/1

== system nucleo_g431re_ihm07m1/SerialReceive/Switch Case Action Subsystem19 ==
  In1 : Inport
  Action Port : ActionPort  ActionPortLabel=case [ 19 ]:
  Data Store Write : DataStoreWrite  DataStoreName=Iq_ref_CL  IndexOptions=Index vector (dialog)  Indices=1  OutputSizes=1
  Saturation : Saturate  LowerLimit=0.05
  wires:
  In1/1 -> Saturation/1
  Saturation/1 -> Data Store Write/1

== system nucleo_g431re_ihm07m1/SerialReceive/Switch Case Action Subsystem2 ==
  In1 : Inport
  Action Port : ActionPort  ActionPortLabel=case [ 2 ]:
  Data Store Write2 : DataStoreWrite  DataStoreName=V_rated  IndexOptions=Index vector (dialog)  Indices=1  OutputSizes=1
  wires:
  In1/1 -> Data Store Write2/1

== system nucleo_g431re_ihm07m1/SerialReceive/Switch Case Action Subsystem20 ==
  In1 : Inport
  Action Port : ActionPort  ActionPortLabel=case [ 20 ]:
  Data Store Write : DataStoreWrite  DataStoreName=under_voltage_limit  IndexOptions=Index vector (dialog)  Indices=1  OutputSizes=1
  Saturation : Saturate  UpperLimit=1  LowerLimit=0.1
  wires:
  In1/1 -> Saturation/1
  Saturation/1 -> Data Store Write/1

== system nucleo_g431re_ihm07m1/SerialReceive/Switch Case Action Subsystem21 ==
  In1 : Inport
  Action Port : ActionPort  ActionPortLabel=case [ 21 ]:
  Data Store Write : DataStoreWrite  DataStoreName=over_current_limit  IndexOptions=Index vector (dialog)  Indices=1  OutputSizes=1
  Saturation : Saturate  UpperLimit=1.2  LowerLimit=0.2
  wires:
  In1/1 -> Saturation/1
  Saturation/1 -> Data Store Write/1

== system nucleo_g431re_ihm07m1/SerialReceive/Switch Case Action Subsystem22 ==
  In1 : Inport
  Action Port : ActionPort  ActionPortLabel=case [ 22 ]:
  Data Store Write1 : DataStoreWrite  DataStoreName=inertia_end_speed  IndexOptions=Index vector (dialog)  Indices=1  OutputSizes=1
  Saturation : Saturate  UpperLimit=0.7  LowerLimit=0.25
  wires:
  In1/1 -> Saturation/1
  Saturation/1 -> Data Store Write1/1

== system nucleo_g431re_ihm07m1/SerialReceive/Switch Case Action Subsystem3 ==
  In1 : Inport
  Action Port : ActionPort  ActionPortLabel=case [ 3 ]:
  Data Store Write4 : DataStoreWrite  DataStoreName=speed_rated  IndexOptions=Index vector (dialog)  Indices=1  OutputSizes=1
  wires:
  In1/1 -> Data Store Write4/1

== system nucleo_g431re_ihm07m1/SerialReceive/Switch Case Action Subsystem4 ==
  In1 : Inport
  Action Port : ActionPort  ActionPortLabel=case [ 4 ]:
  Data Store Write3 : DataStoreWrite  DataStoreName=pole_pairs  IndexOptions=Index vector (dialog)  Indices=1  OutputSizes=1
  wires:
  In1/1 -> Data Store Write3/1

== system nucleo_g431re_ihm07m1/SerialReceive/Switch Case Action Subsystem5 ==
  In1 : Inport
  Action Port : ActionPort  ActionPortLabel=case [ 10 ]:
  Data Store Write3 : DataStoreWrite  DataStoreName=inverter_V_max  IndexOptions=Index vector (dialog)  Indices=1  OutputSizes=1
  wires:
  In1/1 -> Data Store Write3/1

== system nucleo_g431re_ihm07m1/SerialReceive/Switch Case Action Subsystem6 ==
  In1 : Inport
  Action Port : ActionPort  ActionPortLabel=case [ 5 ]:
  Data Store Write3 : DataStoreWrite  DataStoreName=RsMeasTestTime  IndexOptions=Index vector (dialog)  Indices=1  OutputSizes=1
  wires:
  In1/1 -> Data Store Write3/1

== system nucleo_g431re_ihm07m1/SerialReceive/Switch Case Action Subsystem7 ==
  In1 : Inport
  Action Port : ActionPort  ActionPortLabel=case [ 6 ]:
  Data Store Write3 : DataStoreWrite  DataStoreName=R_board  IndexOptions=Index vector (dialog)  Indices=1  OutputSizes=1
  wires:
  In1/1 -> Data Store Write3/1

== system nucleo_g431re_ihm07m1/SerialReceive/Switch Case Action Subsystem8 ==
  In1 : Inport
  Action Port : ActionPort  ActionPortLabel=case [ 7 ]:
  Data Store Write3 : DataStoreWrite  DataStoreName=currentPU_RWV  IndexOptions=Index vector (dialog)  Indices=1  OutputSizes=1
  wires:
  In1/1 -> Data Store Write3/1

== system nucleo_g431re_ihm07m1/SerialReceive/Switch Case Action Subsystem9 ==
  In1 : Inport
  Action Port : ActionPort  ActionPortLabel=case [ 8 ]:
  Data Store Write3 : DataStoreWrite  DataStoreName=sigma  IndexOptions=Index vector (dialog)  Indices=1  OutputSizes=1
  wires:
  In1/1 -> Data Store Write3/1

== system nucleo_g431re_ihm07m1/Alogrithm/Control Algorithm/CurrentScaling1 ==
  IA/IB : Inport
  Add : Sum  Inputs=-+
  Data Store Read : DataStoreRead  DataStoreName=Ia_avg_cal  IndexOptions=Index vector (dialog)  Indices=1  OutputSizes=1
  Data Store Read1 : DataStoreRead  DataStoreName=Ib_avg_cal  IndexOptions=Index vector (dialog)  Indices=1  OutputSizes=1
  Data Type Conversion : DataTypeConversion  OutDataTypeStr=int32  ConvertRealWorld=Stored Integer (SI)  SaturateOnIntegerOverflow=off  RndMeth=Floor
  Data Type Conversion2 : DataTypeConversion  OutDataTypeStr=int32  RndMeth=Simplest  SaturateOnIntegerOverflow=off
  Data Type Conversion3 : DataTypeConversion  OutDataTypeStr=int32  RndMeth=Simplest  SaturateOnIntegerOverflow=off
  Data Type Conversion4 : DataTypeConversion  OutDataTypeStr=single  RndMeth=Simplest  SaturateOnIntegerOverflow=off
  Demux : Demux  Outputs=2
  Mux : Mux  Inputs=2
  count_to_PU : Gain  Commented=on  Gain=-1/(627*inverter.I_max)  OutDataTypeStr=single  RndMeth=Simplest
  count_to_PU1 : Gain  Gain=-1/2048  OutDataTypeStr=single  RndMeth=Simplest
  count_to_PU2 : Gain  OutDataTypeStr=single  RndMeth=Simplest
  Ia : Outport  VectorParamsAs1DForOutWhenUnconnected=off
  Ib : Outport  Port=2  VectorParamsAs1DForOutWhenUnconnected=off
  wires:
  IA/IB/1 -> Data Type Conversion/1
  Mux/1 -> Add/1
  Data Type Conversion/1 -> Add/2
  Add/1 -> Data Type Conversion4/1
  Demux/2 -> Ib/1
  count_to_PU1/1 -> count_to_PU2/1
  Data Store Read1/1 -> Data Type Conversion3/1
  Data Store Read/1 -> Data Type Conversion2/1
  Data Type Conversion3/1 -> Mux/2
  Data Type Conversion4/1 -> count_to_PU1/1
  Demux/1 -> Ia/1
  Data Type Conversion2/1 -> Mux/1
  count_to_PU2/1 -> Demux/1
